simulink model "Passive_and_Active_Cell_Balancing"  (R2022a)
settings: Solver=VariableStepAuto  StartTime=0.0  StopTime=10  RelTol=1e-3
undefined symbols (not defined in the file or in its folder): Ion, Lithium
libraries: spsIdealSwitchLib x7, spsBatteryLib x5, spsSeriesRLCBranchLib x4, spsSeriesRLCLoadLib x3, spsDiodeLib x2, spspowerguiLib x2, spsDCVoltageSourceLib x1, spsGroundLib x1, spsPWMGenerator2LevelLib x1
settings Model: Creator=nikos  LastModifiedBy=nikos

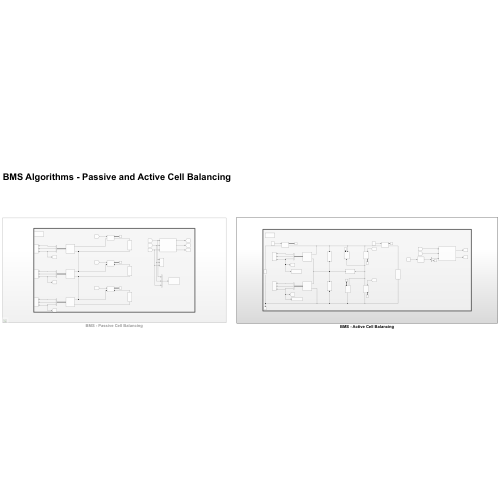
[thumbnail: Simulink's stored preview of the top-level diagram]
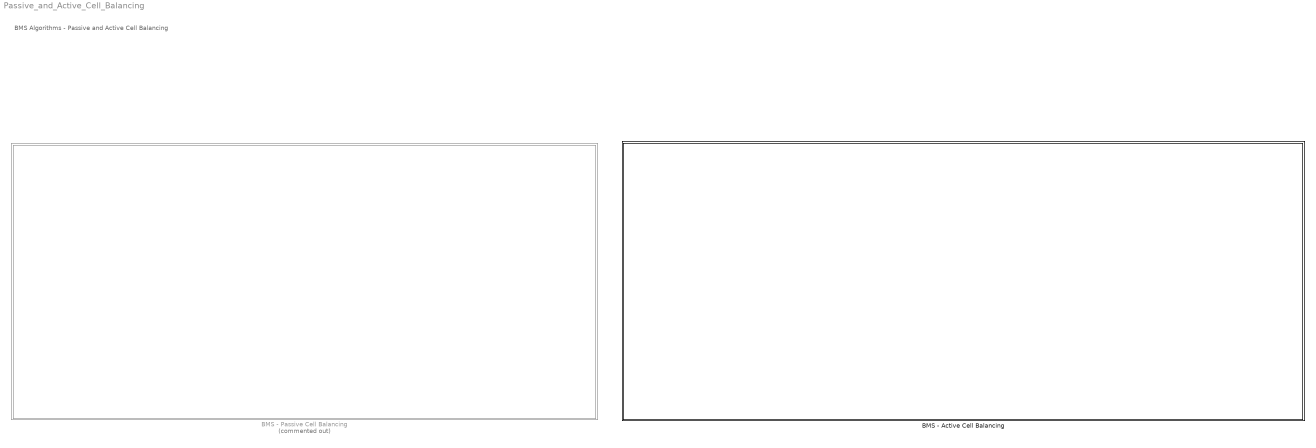
== system Passive_and_Active_Cell_Balancing ==
  note: BMS Algorithms - Passive and Active Cell Balancing
  BMS - Active Cell Balancing : Subsystem
  BMS - Passive Cell Balancing : Subsystem  Commented=on

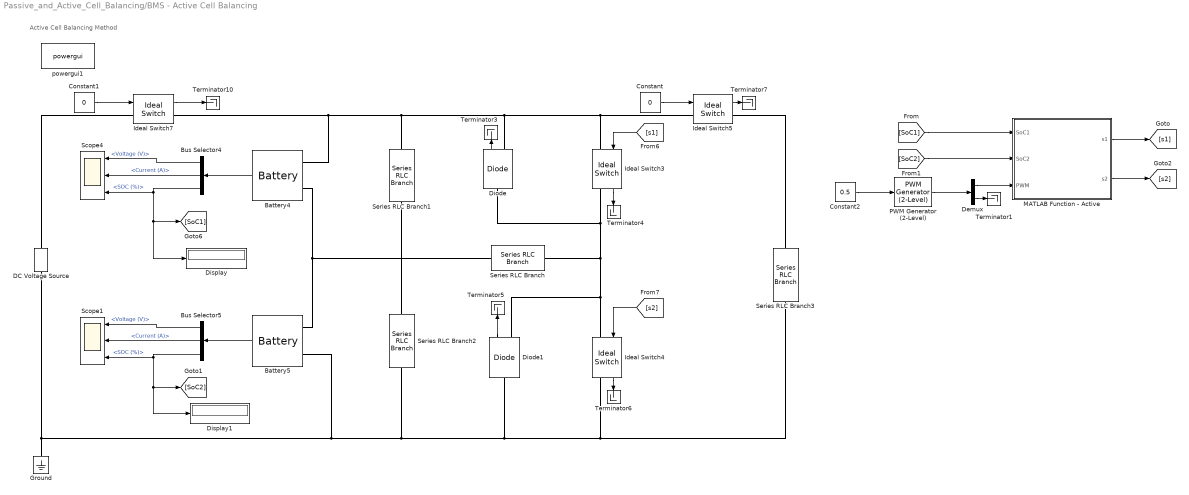
== system Passive_and_Active_Cell_Balancing/BMS - Active Cell Balancing ==
  note: Active Cell Balancing Method
  Battery4 : spsBatteryLib/Battery  BatType=Lithium-Ion  ShowTempParam=off  ThermalPreset=no  ShowAgeParam=off  NomV=3.7  NomQ=4  SOC=60  Batt_Tr=1  PresetModel=on  MaxQ=4  MinV=2.775  FullV=4.3068  Dis_rate=1.7391  R=0.00925  Normal_OP=3.6174  expZone="[3.9974     0.19652]"  current=[6.5 13 32.5]  Units=Time  Tci=20  NomT=20  T2=-30  MaxQ2=4.8  FullV2=7.1  Normal_OP2=5.655  expZone2="[6.58           1]"  Rca=0.6  ti=2000  Dp=0  Neq0=0  Tsim=1e6  Ta1=25  Qeol=5.4*0.9  Reol=0.013333*1.2  Char_age=[2.3478, 3]  Dis_age=[2.3478, 10]  N1=1500  N2=10500  N3=1000  N4=1400  Ta2=45  N5=950
  Battery5 : spsBatteryLib/Battery  BatType=Lithium-Ion  ShowTempParam=off  ThermalPreset=no  ShowAgeParam=off  NomV=3.7  NomQ=4  SOC=35  Batt_Tr=1  PresetModel=on  MaxQ=4  MinV=2.775  FullV=4.3068  Dis_rate=1.7391  R=0.00925  Normal_OP=3.6174  expZone="[3.9974     0.19652]"  current=[6.5 13 32.5]  Units=Time  Tci=20  NomT=20  T2=-30  MaxQ2=4.8  FullV2=7.1  Normal_OP2=5.655  expZone2="[6.58           1]"  Rca=0.6  ti=2000  Dp=0  Neq0=0  Tsim=1e6  Ta1=25  Qeol=5.4*0.9  Reol=0.013333*1.2  Char_age=[2.3478, 3]  Dis_age=[2.3478, 10]  N1=1500  N2=10500  N3=1000  N4=1400  Ta2=45  N5=950
  Bus Selector4 : BusSelector  OutputSignals=Voltage (V),Current (A),SOC (%)
  Bus Selector5 : BusSelector  OutputSignals=Voltage (V),Current (A),SOC (%)
  Constant : Constant  Value=0
  Constant1 : Constant  Value=0
  Constant2 : Constant  Value=0.5
  DC Voltage Source : spsDCVoltageSourceLib/DC Voltage Source  Amplitude=100  Measurements=None
  Demux : Demux  Outputs=2
  Diode : spsDiodeLib/Diode  Ron=0.001  Lon=0  Vf=0.8  IC=0  UseSnubber=0  Rs=500  Cs=250e-9  Measurements=on
  Diode1 : spsDiodeLib/Diode  Ron=0.001  Lon=0  Vf=0.8  IC=0  UseSnubber=0  Rs=500  Cs=250e-9  Measurements=on
  Display : Display
  Display1 : Display
  Ground : spsGroundLib/Ground  LConnTagsString=a
  Ideal Switch{3..5,7} (4 alike) : spsIdealSwitchLib/Ideal Switch  Ron=0.001  Lon=0  IC=0  Rs=1e5  Cs=inf  Measurements=on
  MATLAB Function - Active : MATLAB Function  TreatAsAtomicUnit=on
  PWM Generator (2-Level) : spsPWMGenerator2LevelLib/PWM Generator (2-Level)  ModulatorType=Single-phase half-bridge (2 pulses)  ModulatorMode=Unsynchronized  Fc=500  Pc=0  nF=27  MinMax="[ -1  1 ]"  SamplingTechnique=Natural  ModulatingSignals=off  m=0.8  Freq=60  Phase=0  Ts=0  ShowCarrierOutport=off
  Scope1 : Scope  NumInputPorts=3
  Scope4 : Scope  NumInputPorts=3
  Series RLC Branch : spsSeriesRLCBranchLib/Series RLC Branch  LConnTagsString=__new0  RConnTagsString=__new0  BranchType=L  Resistance=1  Inductance=1e-3  SetiL0=off  InitialCurrent=0  Capacitance=1e-6  Setx0=off  InitialVoltage=0  Measurements=None
  Series RLC Branch1 : spsSeriesRLCBranchLib/Series RLC Branch  LConnTagsString=__new0  RConnTagsString=__new0  BranchType=C  Resistance=1  Inductance=1e-3  SetiL0=off  InitialCurrent=0  Capacitance=1e-6  Setx0=off  InitialVoltage=0  Measurements=None
  Series RLC Branch2 : spsSeriesRLCBranchLib/Series RLC Branch  LConnTagsString=__new0  RConnTagsString=__new0  BranchType=C  Resistance=1  Inductance=1e-3  SetiL0=off  InitialCurrent=0  Capacitance=1e-6  Setx0=off  InitialVoltage=0  Measurements=None
  Series RLC Branch3 : spsSeriesRLCBranchLib/Series RLC Branch  LConnTagsString=__new0  RConnTagsString=__new0  BranchType=R  Resistance=1  Inductance=1e-3  SetiL0=off  InitialCurrent=0  Capacitance=1e-6  Setx0=off  InitialVoltage=0  Measurements=None
  Terminator{1,3..7,10} (7 alike) : Terminator
  powergui1 : spspowerguiLib/powergui  Priority=1  SimulationMode=Discrete  SampleTime=5e-4  frequency=60  Iterations=50  frequencyindice=0  Pbase=100e6  ErrMax=1e-4  UnitsV=kV  UnitsW=MW  buscounter=0  FunctionMessages=off  echomessages=off  EnableUseOfTLC=off  CurrentSourceSwitches=off  DisableSnubberDevices=off  DisableRonSwitches=off  DisableVfSwitches=off  DisplayEquations=off  AutomaticDiscreteSolvers=off  SolverType=Tustin/Backward Euler (TBE)  Interpol=off  ExternalGateDelay=off  methode=off  Ts=100  x0status=blocks  SPID=on  SwTol=0  HookPort=off  NonlinearTolerance=1e-4  nMaxIteration=100  ContinueOnMaxIteration=off  RestoreLinks=warning  ResistiveCurrentMeasurement=off  Frange=[0:2:500]  Ylog=off  Xlog=on  ShowGrid=off  save=off  variable=ZData  structure=0  ZoomFFT=off  StartTime=0.0  cycles=1  DisplayStyle=1  fundamental=60  FreqAxis=off  MaxFrequency=1000  frequencyindicesteady=1  RmsSteady=1  display=off
  wires:
  Diode1/1 -> Terminator5/1
  Bus Selector5/1 -> Scope1/1  "<Voltage (V)>"
  Ideal Switch4/1 -> Terminator6/1
  Bus Selector4/3 -> Display/1, [SoC1], Scope4/3  "<SOC (%)>"
  Ideal Switch5/1 -> Terminator7/1
  Demux/2 -> Terminator1/1
  Constant1/1 -> Ideal Switch7/1
  Bus Selector4/1 -> Scope4/1  "<Voltage (V)>"
  [s2] -> Ideal Switch4/1
  Battery5/1 -> Bus Selector5/1
  Ideal Switch3/1 -> Terminator4/1
  Bus Selector5/3 -> Scope1/3, Display1/1, [SoC2]  "<SOC (%)>"
  Constant2/1 -> PWM Generator (2-Level)/1
  PWM Generator (2-Level)/1 -> Demux/1
  Bus Selector4/2 -> Scope4/2  "<Current (A)>"
  MATLAB Function - Active/1(s1) -> [s1]
  [SoC1] -> MATLAB Function - Active/1(SoC1)
  Ideal Switch7/1 -> Terminator10/1
  [SoC2] -> MATLAB Function - Active/2(SoC2)
  Battery4/1 -> Bus Selector4/1
  Demux/1 -> MATLAB Function - Active/3(PWM)
  Constant/1 -> Ideal Switch5/1
  [s1] -> Ideal Switch3/1
  Diode/1 -> Terminator3/1
  Bus Selector5/2 -> Scope1/2  "<Current (A)>"
  MATLAB Function - Active/2(s2) -> [s2]
  connections:
  Series RLC Branch3/RConn1 -- Ideal Switch4/RConn1 -- Diode1/LConn1 -- Series RLC Branch2/RConn1 -- Battery5/LConn2 -- DC Voltage Source/LConn1 -- Ground/LConn1
  Ideal Switch3/RConn1 -- Diode/LConn1 -- Series RLC Branch/RConn1 -- Diode1/RConn1 -- Ideal Switch4/LConn1
  Battery5/LConn1 -- Series RLC Branch2/LConn1 -- Series RLC Branch/LConn1 -- Series RLC Branch1/RConn1 -- Battery4/LConn2
  Battery4/LConn1 -- Ideal Switch7/RConn1 -- Series RLC Branch1/LConn1 -- Diode/RConn1 -- Ideal Switch3/LConn1 -- Ideal Switch5/LConn1
  DC Voltage Source/RConn1 -- Ideal Switch7/LConn1
  Ideal Switch5/RConn1 -- Series RLC Branch3/LConn1

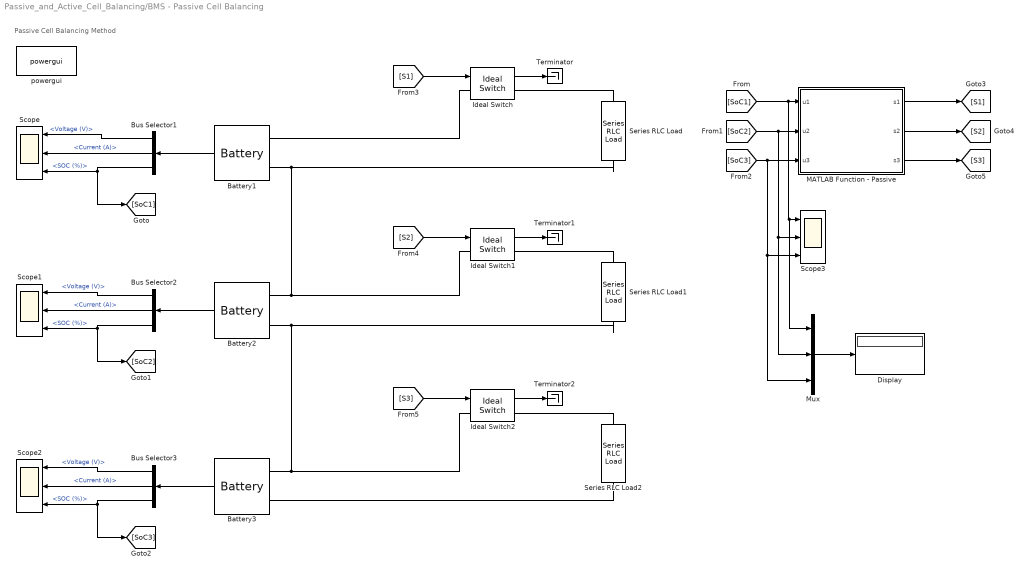
== system Passive_and_Active_Cell_Balancing/BMS - Passive Cell Balancing ==
  note: Passive Cell Balancing Method
  Battery1 : spsBatteryLib/Battery  BatType=Lithium-Ion  ShowTempParam=off  ThermalPreset=no  ShowAgeParam=off  NomV=3.7  NomQ=4  SOC=60  Batt_Tr=1  PresetModel=on  MaxQ=4  MinV=2.775  FullV=4.3068  Dis_rate=1.7391  R=0.00925  Normal_OP=3.6174  expZone="[3.9974     0.19652]"  current=[6.5 13 32.5]  Units=Time  Tci=20  NomT=20  T2=-30  MaxQ2=4.8  FullV2=7.1  Normal_OP2=5.655  expZone2="[6.58           1]"  Rca=0.6  ti=2000  Dp=0  Neq0=0  Tsim=1e6  Ta1=25  Qeol=5.4*0.9  Reol=0.013333*1.2  Char_age=[2.3478, 3]  Dis_age=[2.3478, 10]  N1=1500  N2=10500  N3=1000  N4=1400  Ta2=45  N5=950
  Battery2 : spsBatteryLib/Battery  BatType=Lithium-Ion  ShowTempParam=off  ThermalPreset=no  ShowAgeParam=off  NomV=3.7  NomQ=4  SOC=40  Batt_Tr=1  PresetModel=on  MaxQ=4  MinV=2.775  FullV=4.3068  Dis_rate=1.7391  R=0.00925  Normal_OP=3.6174  expZone="[3.9974     0.19652]"  current=[6.5 13 32.5]  Units=Time  Tci=20  NomT=20  T2=-30  MaxQ2=4.8  FullV2=7.1  Normal_OP2=5.655  expZone2="[6.58           1]"  Rca=0.6  ti=2000  Dp=0  Neq0=0  Tsim=1e6  Ta1=25  Qeol=5.4*0.9  Reol=0.013333*1.2  Char_age=[2.3478, 3]  Dis_age=[2.3478, 10]  N1=1500  N2=10500  N3=1000  N4=1400  Ta2=45  N5=950
  Battery3 : spsBatteryLib/Battery  BatType=Lithium-Ion  ShowTempParam=off  ThermalPreset=no  ShowAgeParam=off  NomV=3.7  NomQ=4  SOC=35  Batt_Tr=1  PresetModel=on  MaxQ=4  MinV=2.775  FullV=4.3068  Dis_rate=1.7391  R=0.00925  Normal_OP=3.6174  expZone="[3.9974     0.19652]"  current=[6.5 13 32.5]  Units=Time  Tci=20  NomT=20  T2=-30  MaxQ2=4.8  FullV2=7.1  Normal_OP2=5.655  expZone2="[6.58           1]"  Rca=0.6  ti=2000  Dp=0  Neq0=0  Tsim=1e6  Ta1=25  Qeol=5.4*0.9  Reol=0.013333*1.2  Char_age=[2.3478, 3]  Dis_age=[2.3478, 10]  N1=1500  N2=10500  N3=1000  N4=1400  Ta2=45  N5=950
  Bus Selector1 : BusSelector  OutputSignals=Voltage (V),Current (A),SOC (%)
  Bus Selector2 : BusSelector  OutputSignals=Voltage (V),Current (A),SOC (%)
  Bus Selector3 : BusSelector  OutputSignals=Voltage (V),Current (A),SOC (%)
  Display : Display
  Ideal Switch : spsIdealSwitchLib/Ideal Switch  Ron=0.001  Lon=0  IC=0  Rs=1e5  Cs=inf  Measurements=on
  Ideal Switch1 : spsIdealSwitchLib/Ideal Switch  Ron=0.001  Lon=0  IC=0  Rs=1e5  Cs=inf  Measurements=on
  Ideal Switch2 : spsIdealSwitchLib/Ideal Switch  Ron=0.001  Lon=0  IC=0  Rs=1e5  Cs=inf  Measurements=on
  MATLAB Function - Passive : MATLAB Function  TreatAsAtomicUnit=on
  Mux : Mux  Inputs=3
  Scope{,1..3} (4 alike) : Scope  NumInputPorts=3
  Series RLC Load : spsSeriesRLCLoadLib/Series RLC Load  LConnTagsString=a  RConnTagsString=__new0  NominalVoltage=4  NominalFrequency=0.1  ActivePower=1e3  InductivePower=0  CapacitivePower=0  Setx0=off  InitialVoltage=0  SetiL0=off  InitialCurrent=0  Measurements=None  LoadType=constant Z
  Series RLC Load1 : spsSeriesRLCLoadLib/Series RLC Load  LConnTagsString=a  RConnTagsString=__new0  NominalVoltage=4  NominalFrequency=0.1  ActivePower=1e3  InductivePower=0  CapacitivePower=0  Setx0=off  InitialVoltage=0  SetiL0=off  InitialCurrent=0  Measurements=None  LoadType=constant Z
  Series RLC Load2 : spsSeriesRLCLoadLib/Series RLC Load  LConnTagsString=a  RConnTagsString=__new0  NominalVoltage=4  NominalFrequency=0.1  ActivePower=1e3  InductivePower=0  CapacitivePower=0  Setx0=off  InitialVoltage=0  SetiL0=off  InitialCurrent=0  Measurements=None  LoadType=constant Z
  Terminator : Terminator
  Terminator1 : Terminator
  Terminator2 : Terminator
  powergui : spspowerguiLib/powergui  Priority=1  SimulationMode=Continuous  SampleTime=50e-6  frequency=60  Iterations=50  frequencyindice=0  Pbase=100e6  ErrMax=1e-4  UnitsV=kV  UnitsW=MW  buscounter=0  FunctionMessages=off  echomessages=off  EnableUseOfTLC=off  CurrentSourceSwitches=off  DisableSnubberDevices=off  DisableRonSwitches=off  DisableVfSwitches=off  DisplayEquations=off  AutomaticDiscreteSolvers=off  SolverType=Tustin/Backward Euler (TBE)  Interpol=off  ExternalGateDelay=off  methode=off  Ts=100  x0status=blocks  SPID=on  SwTol=0  HookPort=off  NonlinearTolerance=1e-4  nMaxIteration=100  ContinueOnMaxIteration=off  RestoreLinks=warning  ResistiveCurrentMeasurement=off  Frange=[0:2:500]  Ylog=off  Xlog=on  ShowGrid=off  save=off  variable=ZData  structure=0  ZoomFFT=off  StartTime=0.0  cycles=1  DisplayStyle=1  fundamental=60  FreqAxis=off  MaxFrequency=1000  frequencyindicesteady=1  RmsSteady=1  display=off
  wires:
  Bus Selector1/3 -> [SoC1], Scope/3  "<SOC (%)>"
  [S3] -> Ideal Switch2/1
  Battery2/1 -> Bus Selector2/1
  Bus Selector2/1 -> Scope1/1  "<Voltage (V)>"
  Mux/1 -> Display/1
  Ideal Switch/1 -> Terminator/1
  Battery3/1 -> Bus Selector3/1
  Ideal Switch1/1 -> Terminator1/1
  Bus Selector1/2 -> Scope/2  "<Current (A)>"
  [SoC1] -> Mux/1, Scope3/1, MATLAB Function - Passive/1(u1)
  Ideal Switch2/1 -> Terminator2/1
  Battery1/1 -> Bus Selector1/1
  MATLAB Function - Passive/3(s3) -> [S3]
  [SoC3] -> Mux/3, Scope3/3, MATLAB Function - Passive/3(u3)
  MATLAB Function - Passive/1(s1) -> [S1]
  Bus Selector2/2 -> Scope1/2  "<Current (A)>"
  [SoC2] -> Mux/2, Scope3/2, MATLAB Function - Passive/2(u2)
  [S2] -> Ideal Switch1/1
  MATLAB Function - Passive/2(s2) -> [S2]
  Bus Selector3/3 -> [SoC3], Scope2/3  "<SOC (%)>"
  Bus Selector3/2 -> Scope2/2  "<Current (A)>"
  Bus Selector3/1 -> Scope2/1  "<Voltage (V)>"
  Bus Selector2/3 -> [SoC2], Scope1/3  "<SOC (%)>"
  Bus Selector1/1 -> Scope/1  "<Voltage (V)>"
  [S1] -> Ideal Switch/1
  connections:
  Ideal Switch2/LConn1 -- Series RLC Load1/RConn1 -- Battery2/LConn2 -- Battery3/LConn1
  Series RLC Load1/LConn1 -- Ideal Switch1/RConn1
  Battery1/LConn2 -- Battery2/LConn1 -- Ideal Switch1/LConn1 -- Series RLC Load/RConn1
  Ideal Switch/LConn1 -- Battery1/LConn1
  Series RLC Load/LConn1 -- Ideal Switch/RConn1
  Series RLC Load2/RConn1 -- Battery3/LConn2
  Series RLC Load2/LConn1 -- Ideal Switch2/RConn1

== matlab function Passive_and_Active_Cell_Balancing/BMS - Active Cell Balancing/MATLAB Function - Active ==
  data: SoC1 input; s1 output; SoC2 input; PWM input; s2 output
function [s1, s2] = fcn(SoC1, SoC2, PWM)

if SoC1 > SoC2
    s1 = PWM;
    s2 = 0;
elseif SoC1 < SoC2
    s2 = PWM
    s1 = 0
else
    s1 = 0
    s2 = 0
end

== matlab function Passive_and_Active_Cell_Balancing/BMS - Passive Cell Balancing/MATLAB Function - Passive ==
  data: u1 input; s1 output; u2 input; u3 input; s2 output; s3 output
function [s1, s2, s3] = fcn(u1, u2, u3)

u1 = int32(u1);
u2 = int32(u2);
u3 = int32(u3);

if ((u1 > u2) || (u1> u3))
    s1 = 1;
else 
    s1 = 0;
end

if ((u2 > u1) || (u2 > u3))
    s2 = 1;
else
    s2 = 0;
end

if ((u3 > u1) || (u3 > u2))
    s3 = 1;
else
    s3 = 0;
end
